simulink model "Deliverable2"  (R2020a)
settings: Solver=FixedStepAuto  StartTime=0.0  StopTime=10.0  FixedStep=1e-3  RelTol=1e-3  EnableMultiTasking=on
undefined symbols (not defined in the file or in its folder): D0, D1, D10, D11, D12, D13, D2, D3, D4, D5, D6, D7, D8, D9, PTA0, PTA1, PTA2, PTB23, PTB9, PTC16, PTC17, PTC2, PTC3, PTC4, PTD0, PTD1, PTD2, PTD3
libraries: frdmk64flib x15
settings Model: ExtModeTrigDuration=5  Creator=haque  LastModifiedBy=haque
settings OptimizationCC: EnhancedBackFolding=on  PassReuseOutputArgsAs=Individual arguments  ZeroExternalMemoryAtStartup=off  ZeroInternalMemoryAtStartup=off  MaxStackSize=64  OptimizeBlockOrder=speed  DifferentSizesBufferReuse=on  OptimizationCustomize=off  EfficientTunableParamExpr=on
settings DebuggingCC: ParameterTunabilityLossMsg=error
settings HardwareCC: ProdBitPerPointer=32  ProdBitPerSizeT=32  ProdBitPerPtrDiffT=32  ProdLargestAtomicInteger=Long  ProdLargestAtomicFloat=Double  ProdWordSize=32  ProdHWDeviceType=ARM Compatible->ARM Cortex
settings SFSimCC: MATLABDynamicMemAlloc=off
settings RTWCC: SystemTargetFile=ert.tlc  HardwareBoard=NXP FRDM-K64F  TemplateMakefile=ert_default_tmf  Toolchain=GNU Tools for ARM Embedded Processors
settings CodeAppCC: ForceParamTrailComments=on  IgnoreCustomStorageClasses=off  OperatorAnnotations=on  SimulinkDataObjDesc=on  SFDataObjDesc=on  InsertBlockDesc=on

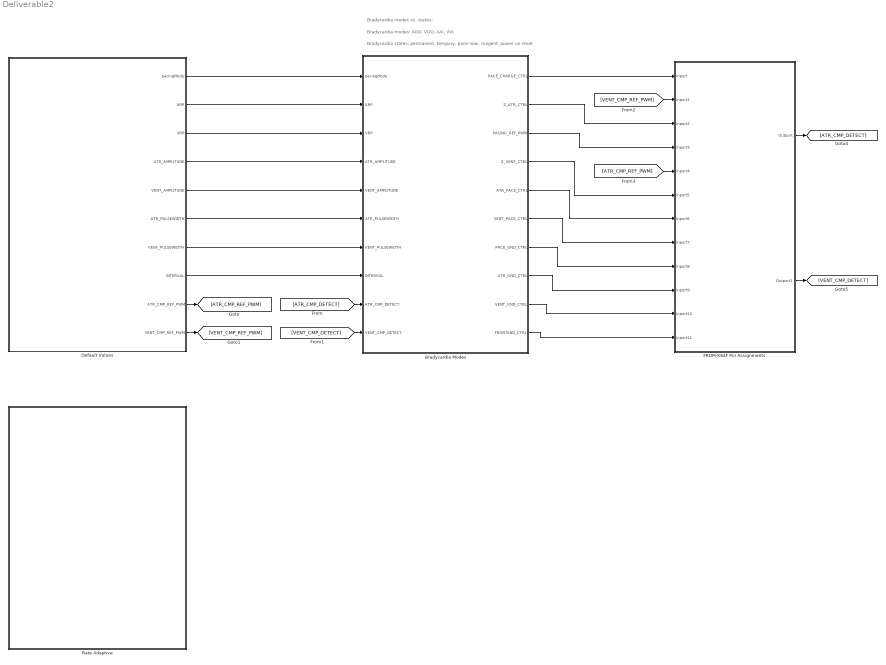
== system Deliverable2 ==
  note: Bradycardia modes vs. states:
  note: Bradycardia states: permanent, tempory, pace now, magent, power on reset
  note: Bradycardia modes: AOO, VOO, AAI, VVI
  Bradycardia Modes : Stateflow chart  TreatAsAtomicUnit=on
  Default Values : Subsystem
  FRDM-K64F Pin Assignments : Subsystem
  Rate Adaptive : Subsystem
  wires:
  Bradycardia Modes/1(PACE_CHARGE_CTRL) -> FRDM-K64F Pin Assignments/1(Inport)
  Bradycardia Modes/2(Z_ATR_CTRL) -> FRDM-K64F Pin Assignments/3(Inport2)
  Bradycardia Modes/3(PACING_REF_PWM) -> FRDM-K64F Pin Assignments/4(Inport3)
  Bradycardia Modes/4(Z_VENT_CTRL) -> FRDM-K64F Pin Assignments/6(Inport5)
  Bradycardia Modes/5(ATR_PACE_CTRL) -> FRDM-K64F Pin Assignments/7(Inport6)
  Bradycardia Modes/6(VENT_PACE_CTRL) -> FRDM-K64F Pin Assignments/8(Inport7)
  Bradycardia Modes/7(PACE_GND_CTRL) -> FRDM-K64F Pin Assignments/9(Inport8)
  Bradycardia Modes/8(ATR_GND_CTRL) -> FRDM-K64F Pin Assignments/10(Inport9)
  Bradycardia Modes/9(VENT_GND_CTRL) -> FRDM-K64F Pin Assignments/11(Inport10)
  Bradycardia Modes/10(FRONTEND_CTRL) -> FRDM-K64F Pin Assignments/12(Inport11)
  Default Values/1(pacingMode) -> Bradycardia Modes/1(pacingMode)
  Default Values/3(VRP) -> Bradycardia Modes/3(VRP)
  Default Values/2(ARP) -> Bradycardia Modes/2(ARP)
  Default Values/6(ATR_PULSEWIDTH) -> Bradycardia Modes/6(ATR_PULSEWIDTH)
  Default Values/8(INTERVAL) -> Bradycardia Modes/8(INTERVAL)
  Default Values/7(VENT_PULSEWIDTH) -> Bradycardia Modes/7(VENT_PULSEWIDTH)
  Default Values/5(VENT_AMPLITUDE) -> Bradycardia Modes/5(VENT_AMPLITUDE)
  Default Values/4(ATR_AMPLITUDE) -> Bradycardia Modes/4(ATR_AMPLITUDE)
  FRDM-K64F Pin Assignments/1(Outport) -> [ATR_CMP_DETECT]
  FRDM-K64F Pin Assignments/2(Outport1) -> [VENT_CMP_DETECT]
  [ATR_CMP_DETECT] -> Bradycardia Modes/9(ATR_CMP_DETECT)
  [VENT_CMP_DETECT] -> Bradycardia Modes/10(VENT_CMP_DETECT)
  [VENT_CMP_REF_PWM] -> FRDM-K64F Pin Assignments/2(Inport1)
  Default Values/9(ATR_CMP_REF_PWM) -> [ATR_CMP_REF_PWM]
  Default Values/10(VENT_CMP_REF_PWM) -> [VENT_CMP_REF_PWM]
  [ATR_CMP_REF_PWM] -> FRDM-K64F Pin Assignments/5(Inport4)

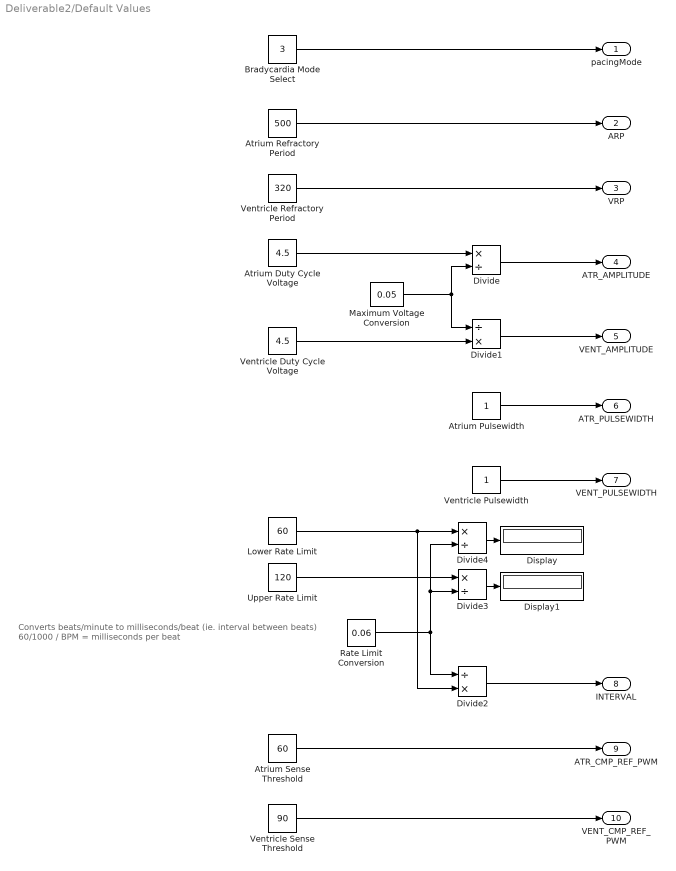
== system Deliverable2/Default Values ==
  note: Converts beats/minute to milliseconds/beat (ie. interval between beats)
      | 60/1000 / BPM = milliseconds per beat
  Atrium Duty Cycle Voltage : Constant  Value=4.5
  Atrium Pulsewidth : Constant
  Atrium Refractory Period : Constant  Value=500
  Atrium Sense Threshold : Constant  Value=60
  Bradycardia Mode Select : Constant  Value=3
  Display : Display
  Display1 : Display
  Divide : Product  Inputs=*/
  Divide1 : Product  Inputs=/*
  Divide2 : Product  Inputs=/*
  Divide3 : Product  Inputs=*/
  Divide4 : Product  Inputs=*/
  Lower Rate Limit : Constant  Value=60
  Maximum Voltage Conversion : Constant  Value=0.05
  Rate Limit Conversion : Constant  Value=0.06
  Upper Rate Limit : Constant  Value=120
  Ventricle Duty Cycle Voltage : Constant  Value=4.5
  Ventricle Pulsewidth : Constant
  Ventricle Refractory Period : Constant  Value=320
  Ventricle Sense Threshold : Constant  Value=90
  pacingMode : Outport
  ARP : Outport  Port=2
  VRP : Outport  Port=3
  ATR_AMPLITUDE : Outport  Port=4
  VENT_AMPLITUDE : Outport  Port=5
  ATR_PULSEWIDTH : Outport  Port=6
  VENT_PULSEWIDTH : Outport  Port=7
  INTERVAL : Outport  Port=8
  ATR_CMP_REF_PWM : Outport  Port=9
  VENT_CMP_REF_PWM : Outport  Port=10
  wires:
  Atrium Duty Cycle Voltage/1 -> Divide/1
  Ventricle Pulsewidth/1 -> VENT_PULSEWIDTH/1
  Bradycardia Mode Select/1 -> pacingMode/1
  Divide2/1 -> INTERVAL/1
  Atrium Refractory Period/1 -> ARP/1
  Ventricle Refractory Period/1 -> VRP/1
  Atrium Pulsewidth/1 -> ATR_PULSEWIDTH/1
  Atrium Sense Threshold/1 -> ATR_CMP_REF_PWM/1
  Ventricle Sense Threshold/1 -> VENT_CMP_REF_PWM/1
  Maximum Voltage Conversion/1 -> Divide1/1, Divide/2
  Divide/1 -> ATR_AMPLITUDE/1
  Divide1/1 -> VENT_AMPLITUDE/1
  Ventricle Duty Cycle Voltage/1 -> Divide1/2
  Upper Rate Limit/1 -> Divide3/1
  Lower Rate Limit/1 -> Divide2/2, Divide4/1
  Divide4/1 -> Display/1
  Divide3/1 -> Display1/1
  Rate Limit Conversion/1 -> Divide3/2, Divide4/2, Divide2/1

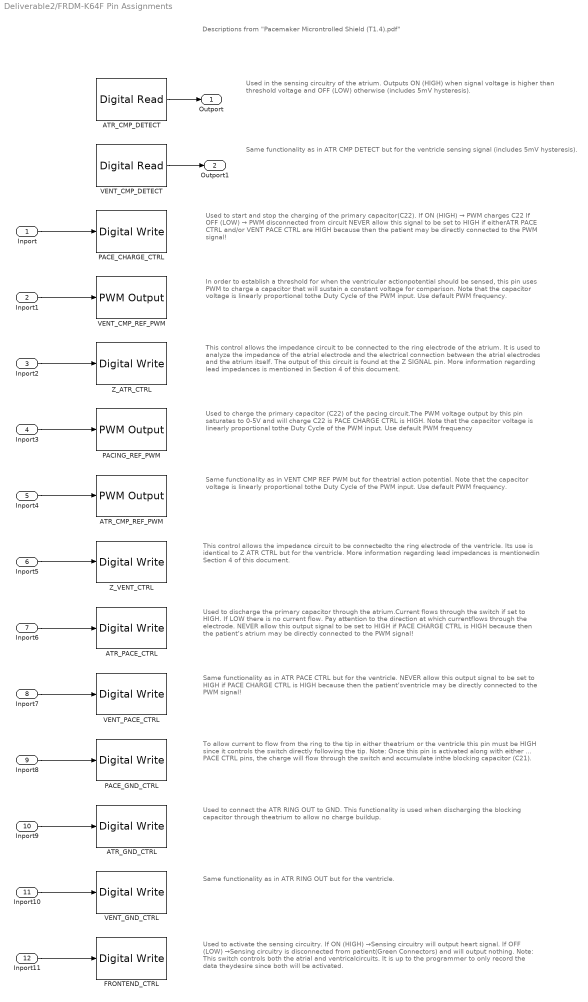
== system Deliverable2/FRDM-K64F Pin Assignments ==
  note: Used to activate the sensing circuitry.
      | If ON (HIGH) →Sensing circuitry will output heart signal.
      | If OFF (LOW) →Sensing circuitry is disconnected from patient(Green Connectors) and will output nothing.
      |
      | Note: This switch controls both the atrial and ventricalcircuits. It is up to the programmer to only record the data theydesire since both will be activated.
  note: Same functionality as in ATR RING OUT but for the ventricle.
  note: This control allows the impedance circuit to be connectedto the ring electrode of the ventricle. Its use is identical to Z ATR CTRL but for the ventricle.
      | More information regarding lead impedances is mentionedin Section 4 of this document.
  note: Same functionality as in VENT CMP REF PWM but for theatrial action potential.
      | Note that the capacitor voltage is linearly proportional tothe Duty Cycle of the PWM input. Use default PWM frequency.
  note: This control allows the impedance circuit to be connected to the ring electrode of the atrium.
      | It is used to analyze the impedance of the atrial electrode and the electrical connection between the atrial electrodes and the atrium itself.
      | The output of this circuit is found at the Z SIGNAL pin. More information regarding lead impedances is mentioned in Section 4 of this document.
  note: Descriptions from "Pacemaker Microntrolled Shield (T1.4).pdf"
  note: In order to establish a threshold for when the ventricular actionpotential should be sensed, this pin uses PWM to charge a capacitor that will sustain a constant voltage for comparison.
      | Note that the capacitor voltage is linearly proportional tothe Duty Cycle of the PWM input. Use default PWM frequency.
  note: Used to charge the primary capacitor (C22) of the pacing circuit.The PWM voltage output by this pin saturates to 0-5V and will charge C22 is PACE CHARGE CTRL is HIGH.
      | Note that the capacitor voltage is linearly proportional tothe Duty Cycle of the PWM input. Use default PWM frequency
  note: Used to start and stop the charging of the primary capacitor(C22).
      | If ON (HIGH) → PWM charges C22
      | If OFF (LOW) → PWM disconnected from circuit
      | NEVER allow this signal to be set to HIGH if eitherATR PACE CTRL and/or VENT PACE CTRL are HIGH because then the patient may be directly connected to the PWM signal!
  note: To allow current to flow from the ring to the tip in either theatrium or the ventricle this pin must be HIGH since it controls the switch directly following the tip.
      | Note: Once this pin is activated along with either ... PACE CTRL pins, the charge will flow through the switch and accumulate inthe blocking capacitor (C21).
  note: Same functionality as in ATR CMP DETECT but for the ventricle sensing signal (includes 5mV hysteresis).
  note: Same functionality as in ATR PACE CTRL but for the ventricle.
      | NEVER allow this output signal to be set to HIGH if PACE CHARGE CTRL is HIGH because then the patient’sventricle may be directly connected to the PWM signal!
  note: Used in the sensing circuitry of the atrium. Outputs ON (HIGH) when signal voltage is higher than threshold voltage and OFF (LOW) otherwise (includes 5mV hysteresis).
  note: Used to discharge the primary capacitor through the atrium.Current flows through the switch if set to HIGH. If LOW there is no current flow. Pay attention to the direction at which currentflows through the electrode.
      | NEVER allow this output signal to be set to HIGH if PACE CHARGE CTRL is HIGH because then the patient’s atrium may be directly connected to the PWM signal!
  note: Used to connect the ATR RING OUT to GND. This functionality is used when discharging the blocking capacitor through theatrium to allow no charge buildup.
  Inport : Inport
  Inport1 : Inport  Port=2
  Inport2 : Inport  Port=3
  Inport3 : Inport  Port=4
  Inport4 : Inport  Port=5
  Inport5 : Inport  Port=6
  Inport6 : Inport  Port=7
  Inport7 : Inport  Port=8
  Inport8 : Inport  Port=9
  Inport9 : Inport  Port=10
  Inport10 : Inport  Port=11
  Inport11 : Inport  Port=12
  ATR_CMP_DETECT : frdmk64flib/Digital Read  Whichpin=PTC16 (D0)  SampleTime=-1
  ATR_CMP_REF_PWM : frdmk64flib/PWM Output  Whichpin=PTC2 (D6)  InitialFrequency=2000  InitialDutyCycle=30
  ATR_GND_CTRL : frdmk64flib/Digital Write  Whichpin=PTD2 (D11)
  ATR_PACE_CTRL : frdmk64flib/Digital Write  Whichpin=PTA0 (D8)
  FRONTEND_CTRL : frdmk64flib/Digital Write  Whichpin=PTD1 (D13)
  PACE_CHARGE_CTRL : frdmk64flib/Digital Write  Whichpin=PTB9 (D2)
  PACE_GND_CTRL : frdmk64flib/Digital Write  Whichpin=PTD0 (D10)
  PACING_REF_PWM : frdmk64flib/PWM Output  Whichpin=PTA2 (D5)  InitialFrequency=2000  InitialDutyCycle=30
  VENT_CMP_DETECT : frdmk64flib/Digital Read  Whichpin=PTC17 (D1)  SampleTime=-1
  VENT_CMP_REF_PWM : frdmk64flib/PWM Output  Whichpin=PTA1 (D3)  InitialFrequency=2000  InitialDutyCycle=30
  VENT_GND_CTRL : frdmk64flib/Digital Write  Whichpin=PTD3 (D12)
  VENT_PACE_CTRL : frdmk64flib/Digital Write  Whichpin=PTC4 (D9)
  Z_ATR_CTRL : frdmk64flib/Digital Write  Whichpin=PTB23 (D4)
  Z_VENT_CTRL : frdmk64flib/Digital Write  Whichpin=PTC3 (D7)
  Outport : Outport
  Outport1 : Outport  Port=2
  wires:
  Inport10/1 -> VENT_GND_CTRL/1
  Inport9/1 -> ATR_GND_CTRL/1
  Inport1/1 -> VENT_CMP_REF_PWM/1
  Inport7/1 -> VENT_PACE_CTRL/1
  Inport2/1 -> Z_ATR_CTRL/1
  Inport8/1 -> PACE_GND_CTRL/1
  Inport3/1 -> PACING_REF_PWM/1
  Inport4/1 -> ATR_CMP_REF_PWM/1
  VENT_CMP_DETECT/1 -> Outport1/1
  Inport5/1 -> Z_VENT_CTRL/1
  Inport11/1 -> FRONTEND_CTRL/1
  Inport6/1 -> ATR_PACE_CTRL/1
  ATR_CMP_DETECT/1 -> Outport/1
  Inport/1 -> PACE_CHARGE_CTRL/1

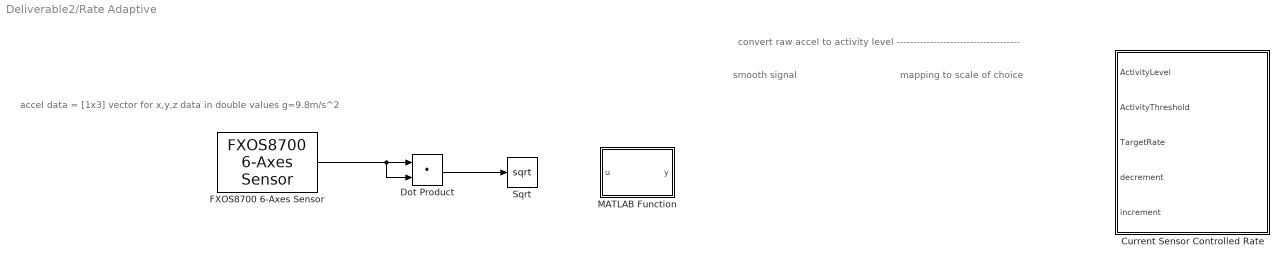
== system Deliverable2/Rate Adaptive ==
  note: accel data = [1x3] vector for x,y,z data in double values g=9.8m/s^2
  note: convert raw accel to activity level -------------------------------------
  note: mapping to scale of choice
  note: smooth signal
  Current Sensor Controlled Rate : Stateflow chart  TreatAsAtomicUnit=on
  Dot Product : DotProduct  InputSameDT=on  OutDataTypeStr=Inherit: Inherit via internal rule
  FXOS8700 6-Axes Sensor : frdmk64flib/FXOS8700 6-Axes Sensor  Activesensor=Accelerometer only  ODR=800Hz  HybridODR=400Hz  Accelfullrange=-4g to +4g  SampleTime=-1
  MATLAB Function : MATLAB Function  TreatAsAtomicUnit=on
  Sqrt : Sqrt  SaturateOnIntegerOverflow=on
  wires:
  FXOS8700 6-Axes Sensor/1 -> Dot Product/2, Dot Product/1
  Dot Product/1 -> Sqrt/1

== stateflow chart Deliverable2/Bradycardia Modes ==
  state AOOR
    state Wait_Charging
      entry:
      %charging C22 (pg.11)
      ATR_PACE_CTRL = 0
      VENT_PACE_CTRL = 0
      PACING_REF_PWM = ATR_AMPLITUDE;  % sets amplitude (duty cycle)
      PACE_CHARGE_CTRL = 1
      %release C21
      PACE_GND_CTRL = 1
      VENT_GND_CTRL = 0
      Z_ATR_CTRL = 0
      Z_VENT_CTRL = 0
      ATR_PACE_CTRL = 0
      ATR_GND_CTRL = 1
      VENT_GND_CTRL = 0
    state Pace_Discharging
      entry:
      %release C22 to charge C21
      PACE_CHARGE_CTRL = 0
      PACE_GND_CTRL = 1
      VENT_PACE_CTRL = 0
      VENT_GND_CTRL = 0
      Z_VENT_CTRL = 0
      Z_ATR_CTRL = 0
      ATR_GND_CTRL = 0
      ATR_PACE_CTRL = 1
    (default) -> AOOR.Wait_Charging
    AOOR.Wait_Charging -> AOOR.Pace_Discharging : [after(INTERVAL, msec)]
    AOOR.Pace_Discharging -> AOOR.Wait_Charging : [after(ATR_PULSEWIDTH,msec)]
  state AOO
    state Wait_Charging
      entry:
      %charging C22 (pg.11)
      ATR_PACE_CTRL = 0
      VENT_PACE_CTRL = 0
      PACING_REF_PWM = ATR_AMPLITUDE;  % sets amplitude (duty cycle)
      PACE_CHARGE_CTRL = 1
      %release C21
      PACE_GND_CTRL = 1
      VENT_GND_CTRL = 0
      Z_ATR_CTRL = 0
      Z_VENT_CTRL = 0
      ATR_PACE_CTRL = 0
      ATR_GND_CTRL = 1
      VENT_GND_CTRL = 0
    state Pace_Discharging
      entry:
      %release C22 to charge C21
      PACE_CHARGE_CTRL = 0
      PACE_GND_CTRL = 1
      VENT_PACE_CTRL = 0
      VENT_GND_CTRL = 0
      Z_VENT_CTRL = 0
      Z_ATR_CTRL = 0
      ATR_GND_CTRL = 0
      ATR_PACE_CTRL = 1
    (default) -> AOO.Wait_Charging
    AOO.Wait_Charging -> AOO.Pace_Discharging : [after(INTERVAL, msec)]
    AOO.Pace_Discharging -> AOO.Wait_Charging : [after(ATR_PULSEWIDTH,msec)]
  state PacingModes
    %chooses a pacing mode
    %{
    defined pacingModes:
    AOO = 0
    VOO = 1
    AAI = 2
    VVI = 3
    %}
  state VOOR
    state Wait_Charging
      entry:
      ATR_PACE_CTRL = 0;
      VENT_PACE_CTRL = 0;
      PACE_CHARGE_CTRL = 1;
      PACING_REF_PWM = VENT_AMPLITUDE;  % sets amplitude (duty cycle)
      PACE_GND_CTRL = 1;
      VENT_GND_CTRL = 1;
      ATR_GND_CTRL = 0;
      Z_ATR_CTRL = 0;
      Z_VENT_CTRL = 0;
    state Pace_Discharging
      entry:
      PACE_GND_CTRL = 1
      VENT_PACE_CTRL = 1
      VENT_GND_CTRL = 0
      Z_VENT_CTRL = 0
      Z_ATR_CTRL = 0
      ATR_GND_CTRL = 0
      ATR_PACE_CTRL = 0
      PACE_CHARGE_CTRL = 0;
    (default) -> VOOR.Wait_Charging
    VOOR.Wait_Charging -> VOOR.Pace_Discharging : [after(INTERVAL, msec)]
    VOOR.Pace_Discharging -> VOOR.Wait_Charging : [after(VENT_PULSEWIDTH, msec)]
  state VOO
    state Wait_Charging
      entry:
      ATR_PACE_CTRL = 0;
      VENT_PACE_CTRL = 0;
      PACE_CHARGE_CTRL = 1;
      PACING_REF_PWM = VENT_AMPLITUDE;  % sets amplitude (duty cycle)
      PACE_GND_CTRL = 1;
      VENT_GND_CTRL = 1;
      ATR_GND_CTRL = 0;
      Z_ATR_CTRL = 0;
      Z_VENT_CTRL = 0;
    state Pace_Discharging
      entry:
      PACE_GND_CTRL = 1
      VENT_PACE_CTRL = 1
      VENT_GND_CTRL = 0
      Z_VENT_CTRL = 0
      Z_ATR_CTRL = 0
      ATR_GND_CTRL = 0
      ATR_PACE_CTRL = 0
      PACE_CHARGE_CTRL = 0;
    (default) -> VOO.Wait_Charging
    VOO.Wait_Charging -> VOO.Pace_Discharging : [after(INTERVAL, msec)]
    VOO.Pace_Discharging -> VOO.Wait_Charging : [after(VENT_PULSEWIDTH, msec)]
  state AAIR
    state Charging_C22_Discharging_C21
      entry:
      % Turn on sensing:
      FRONTEND_CTRL = 1
      %Charging C22 Capacitor:
      ATR_PACE_CTRL = 0
      VENT_PACE_CTRL = 0
      PACING_REF_PWM = ATR_AMPLITUDE
      PACE_CHARGE_CTRL = 1
      %
      % Discharging C21 Capacitor
      PACE_GND_CTRL = 1
      VENT_PACE_CTRL = 0
      Z_ATR_CTRL = 0
      Z_VENT_CTRL = 0
      ATR_PACE_CTRL = 0
      VENT_GND_CTRL = 0
      ATR_GND_CTRL = 1
    state Sensing_Heartbeat
      %after ARP, check sense
    state Discharging_C22_Charging_C21
      %AV Pace
      PACE_CHARGE_CTRL = 0
      PACE_GND_CTRL = 1
      ATR_PACE_CTRL = 0
      ATR_GND_CTRL = 0
      Z_ATR_CTRL = 0
      Z_VENT_CTRL = 0
      VENT_GND_CTRL = 0
      ATR_PACE_CTRL = 1
    (default) -> AAIR.Charging_C22_Discharging_C21
    AAIR.Sensing_Heartbeat -> AAIR.Charging_C22_Discharging_C21 [order 2] : [ATR_CMP_DETECT == 1]
    AAIR.Charging_C22_Discharging_C21 -> AAIR.Sensing_Heartbeat : [after(ARP, msec)]
    AAIR.Sensing_Heartbeat -> AAIR.Discharging_C22_Charging_C21 [order 1] : [after(INTERVAL - ARP, msec)]
    AAIR.Discharging_C22_Charging_C21 -> AAIR.Charging_C22_Discharging_C21 : [after(ATR_PULSEWIDTH, msec)]
  state AAI
    state Charging_C22_Discharging_C21
      entry:
      % Turn on sensing:
      FRONTEND_CTRL = 1
      %Charging C22 Capacitor:
      ATR_PACE_CTRL = 0
      VENT_PACE_CTRL = 0
      PACING_REF_PWM = ATR_AMPLITUDE
      PACE_CHARGE_CTRL = 1
      %
      % Discharging C21 Capacitor
      PACE_GND_CTRL = 1
      VENT_PACE_CTRL = 0
      Z_ATR_CTRL = 0
      Z_VENT_CTRL = 0
      ATR_PACE_CTRL = 0
      VENT_GND_CTRL = 0
      ATR_GND_CTRL = 1
    state Sensing_Heartbeat
      %after ARP, check sense
    state Discharging_C22_Charging_C21
      %AV Pace
      PACE_CHARGE_CTRL = 0
      PACE_GND_CTRL = 1
      ATR_PACE_CTRL = 0
      ATR_GND_CTRL = 0
      Z_ATR_CTRL = 0
      Z_VENT_CTRL = 0
      VENT_GND_CTRL = 0
      ATR_PACE_CTRL = 1
    (default) -> AAI.Charging_C22_Discharging_C21
    AAI.Sensing_Heartbeat -> AAI.Charging_C22_Discharging_C21 [order 2] : [ATR_CMP_DETECT == 1]
    AAI.Charging_C22_Discharging_C21 -> AAI.Sensing_Heartbeat : [after(ARP, msec)]
    AAI.Sensing_Heartbeat -> AAI.Discharging_C22_Charging_C21 [order 1] : [after(INTERVAL - ARP, msec)]
    AAI.Discharging_C22_Charging_C21 -> AAI.Charging_C22_Discharging_C21 : [after(ATR_PULSEWIDTH, msec)]
  state VVIR
    state Charging
      entry:
      % Sensing on:
      FRONTEND_CTRL = 1
      % charging C22 capacitor:
      ATR_PACE_CTRL=0
      VENT_PACE_CTRL=0
      PACING_REF_PWM=VENT_AMPLITUDE
      PACE_CHARGE_CTRL=1
      %
      % Release C21 capacitor charge into ventricle gnd
      PACE_GND_CTRL=1
      VENT_PACE_CTRL=0
      Z_ATR_CTRL=0
      Z_VENT_CTRL=0
      ATR_PACE_CTRL=0
      ATR_GND_CTRL=0
      VENT_GND_CTRL=1
      %
      %
      %{
      Purpose: To charge the main pacing capacitor (C22) to a specific voltage, which determines the pacing pulse amplitude.
      What it does: It connects a PWM signal to the capacitor, allowing it to charge up. It also prepares the output circuit for a ventricular pace by connecting the ventricle tip to ground.
      Key Variables/Pins:
      PACE_CHARGE_CTRL = HIGH: This is the main switch that allows the PWM signal to charge capacitor C22.
      PACING_REF_PWM = VENT_AMPLITUDE: This PWM signal's duty cycle determines the final voltage on the capacitor, and thus the strength (amplitude) of the pace.
      VENT_GND_CTRL = HIGH: Prepares the circuit by connecting the ventricle tip to ground, creating a path for the future pacing current.
      FRONTEND_CTRL = HIGH: Turns on the sensing circuitry so the pacemaker can listen for natural heartbeats even while charging.
      %}
    state Transitioning
      % after ventricle refractory period, check sense
    state Discharging
      entry:
      % Release C22 capacitor charge to charge C21 capacitor
      PACE_CHARGE_CTRL=0
      PACE_GND_CTRL=1
      ATR_PACE_CTRL=0
      ATR_GND_CTRL=0
      Z_VENT_CTRL = 0
      Z_ATR_CTRL = 0
      VENT_GND_CTRL = 0
      VENT_PACE_CTRL = 1
      %
      %
      %{
      - To release the energy from capacitor C22 through the heart creating the pacing pulse.
      - It disconnects the charging circuit and connects the charged capacitor (C22) directly to the ventricle ring electrode.
      - The current flows through the heart to the tip (which is grounded), causing the ventricle to contract.
      %}
    (default) -> VVIR.Charging
    VVIR.Transitioning -> VVIR.Charging [order 2] : [VENT_CMP_DETECT == 1]
    VVIR.Discharging -> VVIR.Charging : [after(VENT_PULSEWIDTH,msec)]
    VVIR.Charging -> VVIR.Transitioning : [after(VRP,msec)]
    VVIR.Transitioning -> VVIR.Discharging [order 1] : [after(INTERVAL-VRP,msec)]
  state VVI
    state Charging
      entry:
      % Sensing on:
      FRONTEND_CTRL = 1
      % charging C22 capacitor:
      ATR_PACE_CTRL=0
      VENT_PACE_CTRL=0
      PACING_REF_PWM=VENT_AMPLITUDE
      PACE_CHARGE_CTRL=1
      %
      % Release C21 capacitor charge into ventricle gnd
      PACE_GND_CTRL=1
      VENT_PACE_CTRL=0
      Z_ATR_CTRL=0
      Z_VENT_CTRL=0
      ATR_PACE_CTRL=0
      ATR_GND_CTRL=0
      VENT_GND_CTRL=1
      %
      %
      %{
      Purpose: To charge the main pacing capacitor (C22) to a specific voltage, which determines the pacing pulse amplitude.
      What it does: It connects a PWM signal to the capacitor, allowing it to charge up. It also prepares the output circuit for a ventricular pace by connecting the ventricle tip to ground.
      Key Variables/Pins:
      PACE_CHARGE_CTRL = HIGH: This is the main switch that allows the PWM signal to charge capacitor C22.
      PACING_REF_PWM = VENT_AMPLITUDE: This PWM signal's duty cycle determines the final voltage on the capacitor, and thus the strength (amplitude) of the pace.
      VENT_GND_CTRL = HIGH: Prepares the circuit by connecting the ventricle tip to ground, creating a path for the future pacing current.
      FRONTEND_CTRL = HIGH: Turns on the sensing circuitry so the pacemaker can listen for natural heartbeats even while charging.
      %}
    state Transitioning
      % after ventricle refractory period, check sense
    state Discharging
      entry:
      % Release C22 capacitor charge to charge C21 capacitor
      PACE_CHARGE_CTRL=0
      PACE_GND_CTRL=1
      ATR_PACE_CTRL=0
      ATR_GND_CTRL=0
      Z_VENT_CTRL = 0
      Z_ATR_CTRL = 0
      VENT_GND_CTRL = 0
      VENT_PACE_CTRL = 1
      %
      %
      %{
      - To release the energy from capacitor C22 through the heart creating the pacing pulse.
      - It disconnects the charging circuit and connects the charged capacitor (C22) directly to the ventricle ring electrode.
      - The current flows through the heart to the tip (which is grounded), causing the ventricle to contract.
      %}
    (default) -> VVI.Charging
    VVI.Transitioning -> VVI.Charging [order 2] : [VENT_CMP_DETECT == 1]
    VVI.Discharging -> VVI.Charging : [after(VENT_PULSEWIDTH,msec)]
    VVI.Charging -> VVI.Transitioning : [after(VRP,msec)]
    VVI.Transitioning -> VVI.Discharging [order 1] : [after(INTERVAL-VRP,msec)]
  (default) -> PacingModes
  PacingModes -> AOO [order 7] : [pacingMode==0]
  PacingModes -> AOOR [order 8] : [pacingMode==4]
  PacingModes -> VOOR [order 5] : [pacingMode==5]
  PacingModes -> VOO [order 1] : [pacingMode==1]
  PacingModes -> AAIR [order 4] : [pacingMode==6]
  PacingModes -> AAI [order 2] : [pacingMode==2]
  PacingModes -> VVI [order 6] : [pacingMode==3]
  PacingModes -> VVIR [order 3] : [pacingMode==7]
  data: PACE_CHARGE_CTRL output; Z_ATR_CTRL output; PACING_REF_PWM output; Z_VENT_CTRL output; pacingMode input; ARP input; VRP input; ATR_AMPLITUDE input; VENT_AMPLITUDE input; ATR_PULSEWIDTH input; VENT_PULSEWIDTH input; INTERVAL input; ATR_CMP_DETECT input; VENT_CMP_DETECT input; ATR_PACE_CTRL output; VENT_PACE_CTRL output; PACE_GND_CTRL output; ATR_GND_CTRL output; VENT_GND_CTRL output; FRONTEND_CTRL output; HIGH local =1; FIRST_CYCLE local

== matlab function Deliverable2/Rate Adaptive/MATLAB Function ==
  data: u input; y output
function y = SignalSmoothing(u)
%{ 
u = original signal --> plot (t, u(t))
y = smoothed signal --> plot (t, y(t))
%} 







y = u;


%{
EXAMPLE FROM MATLAB:
https://www.mathworks.com/help/signal/ug/signal-smoothing.html 

ORIGINAL SIGNAL:

load bostemp
days = (1:31*24)/24;
plot(days, tempC)
axis tight
ylabel("Temperature (\circC)")
xlabel("Time elapsed from Jan 1, 2011 (days)")
title("Logan Airport Dry Bulb Temperature (source: NOAA)")



SMOOTH SIGNAL VIA MOVING AVERAGE FILTER:
hoursPerDay = 24;
coeff24hMA = ones(1, hoursPerDay)/hoursPerDay;

avg24hTempC = filter(coeff24hMA, 1, tempC);
plot(days,[tempC avg24hTempC])
legend("Hourly Temp","24 Hour Average (delayed)","location","best")
ylabel("Temperature (\circC)")
xlabel("Time elapsed from Jan 1, 2011 (days)")
title("Logan Airport Dry Bulb Temperature (source: NOAA)")

%}

== stateflow chart Deliverable2/Rate Adaptive/Current Sensor Controlled Rate ==
  state ChosenRate
    entry:
    AdaptiveRate = LRL
  state Increment
    entry:
    AdaptiveRate = AdaptiveRate + increment
  state TargetRate
    % desired heart rate has been achieved
  state Decrement
    entry:
    AdaptiveRate = AdaptiveRate - decrement
  Increment -> Increment [order 2] : after(1000,msec)[ActivityLevel > ActivityThreshold]
  (default) -> ChosenRate
  ChosenRate -> ChosenRate [order 2] : [ActivityLevel < ActivityThreshold]
  ChosenRate -> Increment [order 1] : [ActivityLevel > ActivityThreshold]
  Increment -> TargetRate [order 1] : [AdaptiveRate >= TargetRate]
  Decrement -> ChosenRate [order 3] : [AdaptiveRate <= LRL]
  Decrement -> Increment [order 1] : after(1000,msec)[ActivityLevel > ActivityThreshold]
  Increment -> Decrement [order 3] : after(1000,msec)[ActivityLevel < ActivityThreshold]
  TargetRate -> Decrement : [ActivityLevel < ActivityThreshold]
  Decrement -> Decrement [order 2] : after(1000,msec)[ActivityLevel<ActivityThreshold]
  data: ActivityLevel input; ActivityThreshold input; TargetRate input; decrement input; increment input; AdaptiveRate local; LRL parameter
